simulink model "waves"  (R2018a)
settings: Solver=FixedStepAuto  StartTime=0.0  StopTime=1  FixedStep=1e-6  RelTol=1e-3
libraries: simulink x1
settings Model: Creator=Bhaskar  LastModifiedBy=Bhaskar

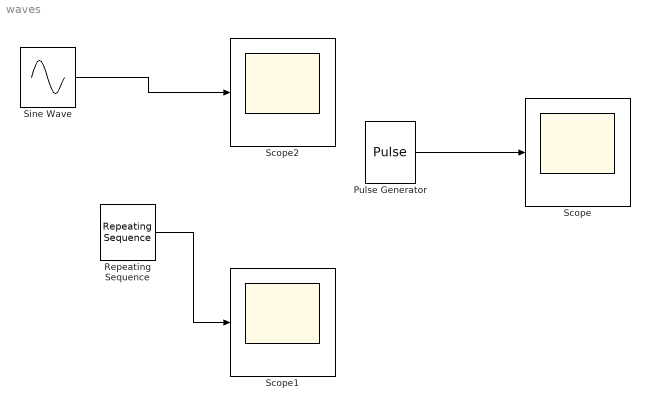
== system waves ==
  Pulse Generator : DiscretePulseGenerator  PulseType=Time based  Period=1/50  PulseWidth=50
  Repeating Sequence : simulink/Sources/Repeating Sequence  rep_seq_t=[0 .25 .5 .75 1]*20e-3  rep_seq_y=[0 1 0 -1 0]
  Scope : Scope
  Scope1 : Scope
  Scope2 : Scope
  Sine Wave : Sin  Frequency=2*pi*50  SampleTime=0
  wires:
  Pulse Generator/1 -> Scope/1
  Repeating Sequence/1 -> Scope1/1
  Sine Wave/1 -> Scope2/1
